simulink model "cart_pendulum_discrete_plants"  (R2018b)
settings: Solver=FixedStepDiscrete  StartTime=0.0  StopTime=2  FixedStep=1e-4  RelTol=1e-3
model workspace (MAT data in the model file):
  Az = [1  9.99990909146e-05  1.33635557195e-08  4.45452527614e-13; 0  0.999981818347  0.000267270311425  1.33635557195e-08; 0  -2.27271355774e-09  1.00000015591  0.000100000005197; 0  -4.54541345962e-05  0.00311817590589  1.00000015591]
  Bz = [9.09085404536e-09; 0.00018181653096; 2.27271355774e-08; 0.000454541345962]
  I = 0.006
  M = 0.5
  Ts = 0.0001
  b = 0.1
  g = 9.8
  l = 0.3
  m = 0.2
  z0 = [0; 0; 0.0872664625997; 0]
settings Model: Creator=volka  LastModifiedBy=volka
settings DataIOCC: ReturnWorkspaceOutputs=on

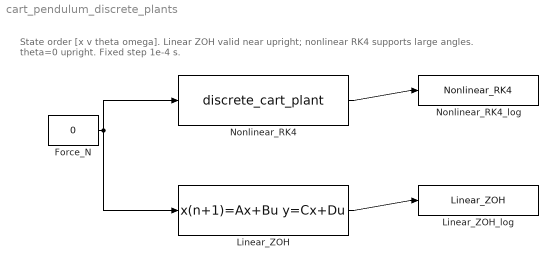
== system cart_pendulum_discrete_plants ==
  note: State order [x v theta omega]. Linear ZOH valid near upright; nonlinear RK4 supports large angles. theta=0 upright. Fixed step 1e-4 s.
  Force_N : Constant  Value=0  SampleTime=Ts
  Linear_ZOH : DiscreteStateSpace  A=Az  B=Bz  C=eye(4)  D=zeros(4,1)  InitialCondition=z0  SampleTime=Ts
  Linear_ZOH_log : ToWorkspace  VariableName=Linear_ZOH  SaveFormat=Structure With Time  SampleTime=-1
  Nonlinear_RK4 : S-Function  FunctionName=discrete_cart_plant  Parameters=Ts,z0,M,m,b,l,I,g  SFunctionDeploymentMode=off  EnableBusSupport=off
  Nonlinear_RK4_log : ToWorkspace  VariableName=Nonlinear_RK4  SaveFormat=Structure With Time  SampleTime=-1
  wires:
  Force_N/1 -> Nonlinear_RK4/1, Linear_ZOH/1
  Nonlinear_RK4/1 -> Nonlinear_RK4_log/1
  Linear_ZOH/1 -> Linear_ZOH_log/1
